simulink model "Aufgabe2_4"  (Simulink 9.1)
settings: Solver=VariableStepAuto  StartTime=0.0  StopTime=10.0  RelTol=1e-3
InitFcn:
  | run('Auf2_1_Initialisierung.m') % Initialisierung
values from neighbouring files (symbols this model uses):
  b1 = 2.39e6    (= 2390000)    [Auf2_1_Initialisierung.m]
  coe = 36.5e6    (= 36500000)    [Auf2_1_Initialisierung.m]
  cp = 75e6    (= 75000000)    [Auf2_1_Initialisierung.m]
  KM = 1/63000    (= 1.5873015873e-05)    [Auf2_1_Initialisierung.m]
  mg = mp + mk    (= 268.7)    [Auf2_1_Initialisierung.m]
libraries: simulink x1
settings Model: Creator=kleist  LastModifiedBy=kleist
settings DataIOCC: SaveFormat=Dataset
settings OptimizationCC: LifeSpan=auto
settings DebuggingCC: UnderspecifiedInitializationDetection=Simplified  MergeDetectMultiDrivingBlocksExec=error  SFUnexpectedBacktrackingDiag=error  SFNoUnconditionalDefaultTransitionDiag=error  SFExecutionAtInitializationDiag=warning
settings HardwareCC: ProdBitPerPointer=64  ProdBitPerSizeT=64  ProdBitPerPtrDiffT=64  ProdLargestAtomicFloat=Float  ProdIntDivRoundTo=Zero  ProdEndianess=LittleEndian  ProdWordSize=64  ProdHWDeviceType=Intel->x86-64 (Windows64)
settings ModelReferenceCC: PropagateSignalLabelsOutOfModel=on
settings CodeAppCC: StateflowObjectComments=off
settings GRTTargetCC: TargetLangStandard=C99 (ISO)  CombineOutputUpdateFcns=on  GRTInterface=off
settings ConfigComp: CovMetricSettings=dwe  CovHtmlReporting=off  CovSaveCumulativeToWorkspaceVar=off  CovSaveSingleToWorkspaceVar=off  CovExternalEMLEnable=on

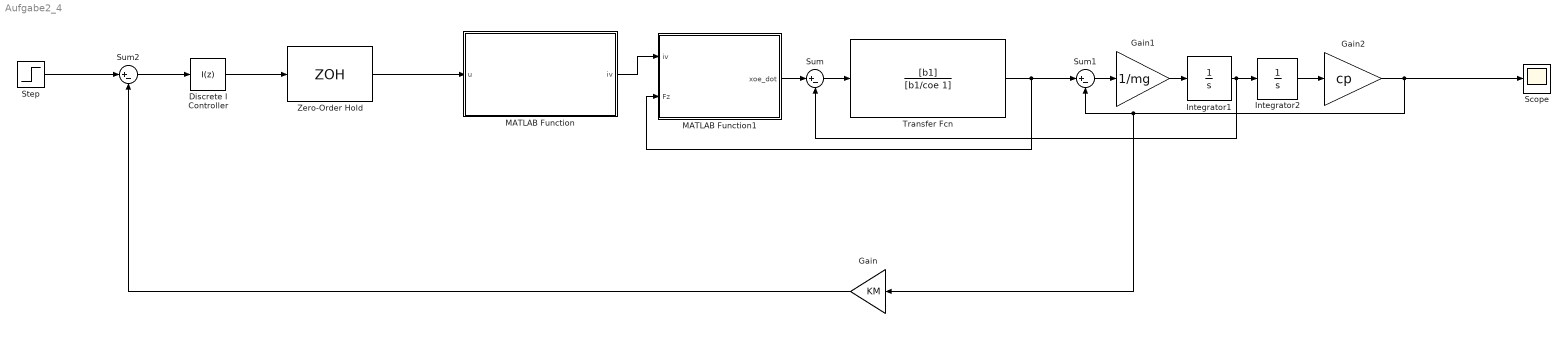
== system Aufgabe2_4 ==
  Discrete I Controller : simulink/Continuous/PID Controller  Controller=I  TimeDomain=Discrete-time  SampleTime=0.015  IntegratorMethod=Forward Euler  FilterMethod=Forward Euler  Form=Parallel  UseFilter=on  ControllerParametersSource=internal  P=0  I=0.273  D=0  N=100  InitialConditionSource=internal  InitialConditionForIntegrator=0  InitialConditionForFilter=0  ExternalReset=none  LimitOutput=off  UpperSaturationLimit=inf  LowerSaturationLimit=-inf  LinearizeAsGain=off  AntiWindupMode=none  Kb=1  TrackingMode=off  Kt=1  PParamMin=[]  PParamMax=[]  IParamMin=[]  IParamMax=[]  DParamMin=[]  DParamMax=[]  NParamMin=[]  NParamMax=[]  KbParamMin=[]  KbParamMax=[]  KtParamMin=[]  KtParamMax=[]  POutMin=[]  POutMax=[]  IOutMin=[]  IOutMax=[]  DOutMin=[]  DOutMax=[]  NOutMin=[]  NOutMax=[]  KbOutMin=[]  KbOutMax=[]  KtOutMin=[]  KtOutMax=[]  IntegratorOutMin=[]  IntegratorOutMax=[]  FilterOutMin=[]  FilterOutMax=[]  SumOutMin=[]  SumOutMax=[]  SumI1OutMin=[]  SumI1OutMax=[]  SumI2OutMin=[]  SumI2OutMax=[]  SumI3OutMin=[]  SumI3OutMax=[]  SumDOutMin=[]  SumDOutMax=[]  SaturationOutMin=[]  SaturationOutMax=[]  IntegratorContinuousStateAttributes=''  IntegratorStateMustResolveToSignalObject=off  IntegratorRTWStateStorageClass=Auto  FilterContinuousStateAttributes=''  FilterStateMustResolveToSignalObject=off  FilterRTWStateStorageClass=Auto  DifferentiatorICPrevScaledInput=0  DifferentiatorOutMin=[]  DifferentiatorOutMax=[]  FilterDiffOutCoefMin=[]  FilterDiffOutCoefMax=[]  SumDenOutMin=[]  SumDenOutMax=[]  SumNumOutMin=[]  SumNumOutMax=[]  ReciprocalOutMin=[]  ReciprocalOutMax=[]  DivideOutMin=[]  DivideOutMax=[]  TunerSelectOption=Transfer Function Based (PID Tuner App)
  Gain : Gain  Gain=KM
  Gain1 : Gain  Gain=1/mg
  Gain2 : Gain  Gain=cp
  Integrator1 : Integrator
  Integrator2 : Integrator
  MATLAB Function : MATLAB Function  TreatAsAtomicUnit=on
  MATLAB Function1 : MATLAB Function  TreatAsAtomicUnit=on
  Scope : Scope
  Step : Step  Time=0  After=0.1  SampleTime=0
  Sum : Sum  Inputs=|+-
  Sum1 : Sum  Inputs=|+-
  Sum2 : Sum  Inputs=|+-
  Transfer Fcn : TransferFcn  Numerator=[b1]  Denominator=[b1/coe 1]
  Zero-Order Hold : ZeroOrderHold  SampleTime=0.015
  wires:
  Discrete I Controller/1 -> Zero-Order Hold/1
  Zero-Order Hold/1 -> MATLAB Function/1(u)
  Sum1/1 -> Gain1/1
  Integrator2/1 -> Gain2/1
  Gain2/1 -> Scope/1, Gain/1, Sum1/2
  Transfer Fcn/1 -> Sum1/1, MATLAB Function1/2(Fz)
  Integrator1/1 -> Sum/2, Integrator2/1
  Sum/1 -> Transfer Fcn/1
  MATLAB Function/1(iv) -> MATLAB Function1/1(iv)
  MATLAB Function1/1(xoe_dot) -> Sum/1
  Gain1/1 -> Integrator1/1
  Step/1 -> Sum2/1
  Gain/1 -> Sum2/2
  Sum2/1 -> Discrete I Controller/1

== matlab function MATLAB Function1 ==
  data: iv input double; xoe_dot output double; Fz input double
function xoe_dot = fcn(iv,Fz)
Ksv = 0.796;%[m/As]
FN = 63000;%[N]
A = 1-Fz/FN*sign(iv);
if A > 0
    xoe_dot = iv*Ksv*sqrt(A);
else
    xoe_dot = 0;
end

== matlab function MATLAB Function ==
  settings: updateMethod=DISCRETE
  data: u input double; iv output double
function iv = fcn(u)
Kl = 1; %[A/V]
ivmax = 1;%[A]
if u>1
    iv = ivmax;
elseif u>=-1 &&u<=1
    iv = Kl*u;
else
    iv = -ivmax;
end
